simulink model "Mrinal_230929228_Simulink"  (R2025a)
settings: Solver=VariableStepAuto  StartTime=0.0  StopTime=40  RelTol=1e-3
libraries: spsSeriesRLCBranchLib x13, spsDCVoltageSourceLib x5, spsGroundLib x3, spsCurrentMeasurementLib x2, spsVoltageMeasurementLib x2, sps_lib x2
settings Model: Creator=MRINAL  LastModifiedBy=MRINAL

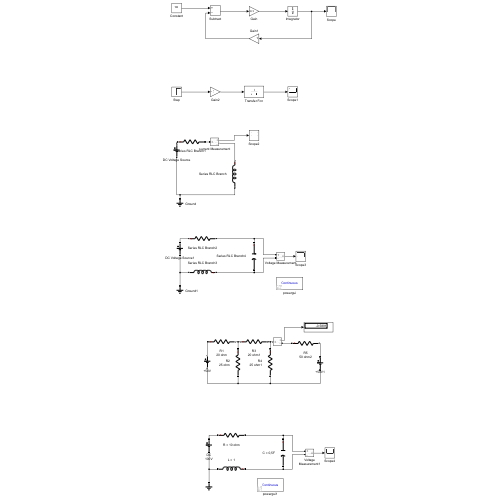
[thumbnail: Simulink's stored preview of the top-level diagram]
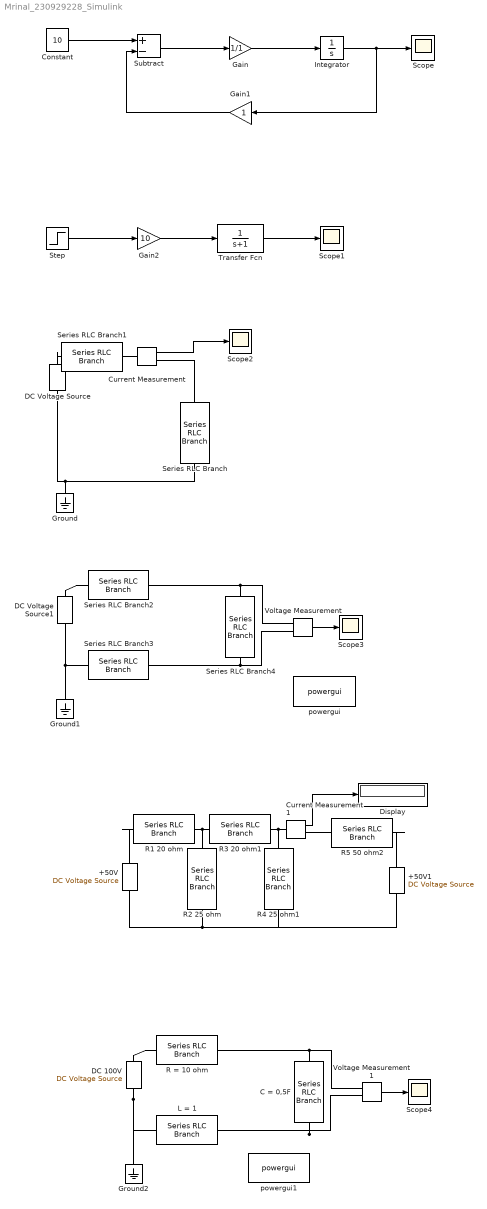
== system Mrinal_230929228_Simulink ==
  +50V : spsDCVoltageSourceLib/DC Voltage Source  Amplitude=50  Measurements=None
  +50V1 : spsDCVoltageSourceLib/DC Voltage Source  Amplitude=50  Measurements=None
  C = 0,5F : spsSeriesRLCBranchLib/Series RLC Branch  LConnTagsString=__new0  RConnTagsString=__new0  BranchType=C  Resistance=1  Inductance=1  SetiL0=off  InitialCurrent=0  Capacitance=0.5  Setx0=off  InitialVoltage=0  Measurements=None
  Constant : Constant  Value=10
  Current Measurement : spsCurrentMeasurementLib/Current Measurement  PhasorSimulation=off  OutputType=Complex  PSBequivalent=0
  Current Measurement1 : spsCurrentMeasurementLib/Current Measurement  PhasorSimulation=off  OutputType=Complex  PSBequivalent=0
  DC 100V : spsDCVoltageSourceLib/DC Voltage Source  Amplitude=100  Measurements=None
  DC Voltage Source : spsDCVoltageSourceLib/DC Voltage Source  Amplitude=10  Measurements=None
  DC Voltage Source1 : spsDCVoltageSourceLib/DC Voltage Source  Amplitude=10  Measurements=None
  Display : Display
  Gain : Gain  Gain=1/1
  Gain1 : Gain
  Gain2 : Gain  Gain=10
  Ground : spsGroundLib/Ground  LConnTagsString=a
  Ground1 : spsGroundLib/Ground  LConnTagsString=a
  Ground2 : spsGroundLib/Ground  LConnTagsString=a
  Integrator : Integrator
  L = 1 : spsSeriesRLCBranchLib/Series RLC Branch  LConnTagsString=__new0  RConnTagsString=__new0  BranchType=L  Resistance=1  Inductance=1  SetiL0=off  InitialCurrent=0  Capacitance=1e-6  Setx0=off  InitialVoltage=0  Measurements=None
  R = 10 ohm : spsSeriesRLCBranchLib/Series RLC Branch  LConnTagsString=__new0  RConnTagsString=__new0  BranchType=R  Resistance=1.23  Inductance=1e-3  SetiL0=off  InitialCurrent=0  Capacitance=1e-6  Setx0=off  InitialVoltage=0  Measurements=None
  R1 20 ohm : spsSeriesRLCBranchLib/Series RLC Branch  LConnTagsString=__new0  RConnTagsString=__new0  BranchType=R  Resistance=20  Inductance=1e-3  SetiL0=off  InitialCurrent=0  Capacitance=1e-6  Setx0=off  InitialVoltage=0  Measurements=None
  R2 25 ohm : spsSeriesRLCBranchLib/Series RLC Branch  LConnTagsString=__new0  RConnTagsString=__new0  BranchType=R  Resistance=25  Inductance=1e-3  SetiL0=off  InitialCurrent=0  Capacitance=1e-6  Setx0=off  InitialVoltage=0  Measurements=None
  R3 20 ohm1 : spsSeriesRLCBranchLib/Series RLC Branch  LConnTagsString=__new0  RConnTagsString=__new0  BranchType=R  Resistance=20  Inductance=1e-3  SetiL0=off  InitialCurrent=0  Capacitance=1e-6  Setx0=off  InitialVoltage=0  Measurements=None
  R4 25 ohm1 : spsSeriesRLCBranchLib/Series RLC Branch  LConnTagsString=__new0  RConnTagsString=__new0  BranchType=R  Resistance=25  Inductance=1e-3  SetiL0=off  InitialCurrent=0  Capacitance=1e-6  Setx0=off  InitialVoltage=0  Measurements=None
  R5 50 ohm2 : spsSeriesRLCBranchLib/Series RLC Branch  LConnTagsString=__new0  RConnTagsString=__new0  BranchType=R  Resistance=50  Inductance=1e-3  SetiL0=off  InitialCurrent=0  Capacitance=1e-6  Setx0=off  InitialVoltage=0  Measurements=None
  Scope{,1..4} (5 alike) : Scope
      Scope settings: Title=230929228_Mrinal_Kumar  ActiveDisplayYMinimum=-1  ActiveDisplayYMaximum=1  YLabel=Current
      Scope1 settings: Title=230929228_Mrinal_Kumar  ActiveDisplayYMinimum=-1.2498457375731515  ActiveDisplayYMaximum=11.248611638158366  YLabel=Current
      Scope2 settings: Title=230929228_Mrinal_Kumar  ActiveDisplayYMinimum=-1  ActiveDisplayYMaximum=1  DataLoggingVariableName=ScopeData2
      Scope3 settings: Title=230929228_Mrinal_Kumar  ActiveDisplayYMinimum=-1.2499701795989464  ActiveDisplayYMaximum=11.24973161639052  YLabel=Voltage (V)  DataLoggingVariableName=ScopeData3
      Scope4 settings: Title=230929228_Mrinal_Kumar  ActiveDisplayYMinimum=-14.98597735302806  ActiveDisplayYMaximum=134.87379617725259  YLabel=Voltage (V)  DataLoggingVariableName=ScopeData4
  Series RLC Branch : spsSeriesRLCBranchLib/Series RLC Branch  LConnTagsString=__new0  RConnTagsString=__new0  BranchType=L  Resistance=1  Inductance=1  SetiL0=off  InitialCurrent=0  Capacitance=1e-6  Setx0=off  InitialVoltage=0  Measurements=None
  Series RLC Branch1 : spsSeriesRLCBranchLib/Series RLC Branch  LConnTagsString=__new0  RConnTagsString=__new0  BranchType=R  Resistance=1  Inductance=1e-3  SetiL0=off  InitialCurrent=0  Capacitance=1e-6  Setx0=off  InitialVoltage=0  Measurements=None
  Series RLC Branch2 : spsSeriesRLCBranchLib/Series RLC Branch  LConnTagsString=__new0  RConnTagsString=__new0  BranchType=R  Resistance=4  Inductance=1e-3  SetiL0=off  InitialCurrent=0  Capacitance=1e-6  Setx0=off  InitialVoltage=0  Measurements=None
  Series RLC Branch3 : spsSeriesRLCBranchLib/Series RLC Branch  LConnTagsString=__new0  RConnTagsString=__new0  BranchType=L  Resistance=1  Inductance=1  SetiL0=off  InitialCurrent=0  Capacitance=1e-6  Setx0=off  InitialVoltage=0  Measurements=None
  Series RLC Branch4 : spsSeriesRLCBranchLib/Series RLC Branch  LConnTagsString=__new0  RConnTagsString=__new0  BranchType=C  Resistance=1  Inductance=1  SetiL0=off  InitialCurrent=0  Capacitance=1  Setx0=off  InitialVoltage=0  Measurements=None
  Step : Step  SampleTime=0
  Subtract : Sum  Inputs=+-
  Transfer Fcn : TransferFcn  Denominator=[1 1]
  Voltage Measurement1 : spsVoltageMeasurementLib/Voltage Measurement  PhasorSimulation=off  OutputType=Complex  PSBequivalent=0
  Voltage Measurement : spsVoltageMeasurementLib/Voltage Measurement  PhasorSimulation=off  OutputType=Complex  PSBequivalent=0
  powergui : sps_lib/powergui  Priority=1  SimulationMode=Continuous  SampleTime=50e-6  frequency=60  Iterations=50  frequencyindice=0  Pbase=100e6  ErrMax=1e-4  UnitsV=kV  UnitsW=MW  buscounter=0  FunctionMessages=off  echomessages=off  EnableUseOfTLC=off  CurrentSourceSwitches=off  DisableSnubberDevices=off  DisableRonSwitches=off  DisableVfSwitches=off  DisplayEquations=off  AutomaticDiscreteSolvers=off  SolverType=Tustin/Backward Euler (TBE)  Interpol=off  ExternalGateDelay=off  methode=off  Ts=100  x0status=zero  SPID=on  SwTol=0  HookPort=off  NonlinearTolerance=1e-4  nMaxIteration=100  ContinueOnMaxIteration=off  RestoreLinks=warning  ResistiveCurrentMeasurement=off  Frange=[0:2:500]  Ylog=off  Xlog=on  ShowGrid=off  save=off  variable=ZData  structure=0  ZoomFFT=off  StartTime=0.0  cycles=1  DisplayStyle=1  fundamental=60  FreqAxis=off  MaxFrequency=1000  frequencyindicesteady=1  RmsSteady=1  display=off
  powergui1 : sps_lib/powergui  Priority=1  SimulationMode=Continuous  SampleTime=50e-6  frequency=60  Iterations=50  frequencyindice=0  Pbase=100e6  ErrMax=1e-4  UnitsV=kV  UnitsW=MW  buscounter=0  FunctionMessages=off  echomessages=off  EnableUseOfTLC=off  CurrentSourceSwitches=off  DisableSnubberDevices=off  DisableRonSwitches=off  DisableVfSwitches=off  DisplayEquations=off  AutomaticDiscreteSolvers=off  SolverType=Tustin/Backward Euler (TBE)  Interpol=off  ExternalGateDelay=off  methode=off  Ts=100  x0status=zero  SPID=on  SwTol=0  HookPort=off  NonlinearTolerance=1e-4  nMaxIteration=100  ContinueOnMaxIteration=off  RestoreLinks=warning  ResistiveCurrentMeasurement=off  Frange=[0:2:500]  Ylog=off  Xlog=on  ShowGrid=off  save=off  variable=ZData  structure=0  ZoomFFT=off  StartTime=0.0  cycles=1  DisplayStyle=1  fundamental=60  FreqAxis=off  MaxFrequency=1000  frequencyindicesteady=1  RmsSteady=1  display=off
  wires:
  Constant/1 -> Subtract/1
  Subtract/1 -> Gain/1
  Gain/1 -> Integrator/1
  Integrator/1 -> Gain1/1, Scope/1
  Gain1/1 -> Subtract/2
  Step/1 -> Gain2/1
  Gain2/1 -> Transfer Fcn/1
  Transfer Fcn/1 -> Scope1/1
  Current Measurement/1 -> Scope2/1
  Voltage Measurement/1 -> Scope3/1
  Current Measurement1/1 -> Display/1
  Voltage Measurement1/1 -> Scope4/1
  connections:
  Current Measurement/RConn1 -- Series RLC Branch/LConn1
  Series RLC Branch/RConn1 -- DC Voltage Source/LConn1 -- Ground/LConn1
  DC Voltage Source/RConn1 -- Series RLC Branch1/LConn1
  Series RLC Branch1/RConn1 -- Current Measurement/LConn1
  Ground1/LConn1 -- Series RLC Branch3/RConn1 -- DC Voltage Source1/LConn1
  Series RLC Branch2/LConn1 -- DC Voltage Source1/RConn1
  Series RLC Branch4/LConn1 -- Series RLC Branch2/RConn1 -- Voltage Measurement/LConn1
  Series RLC Branch3/LConn1 -- Voltage Measurement/LConn2 -- Series RLC Branch4/RConn1
  R3 20 ohm1/LConn1 -- R2 25 ohm/LConn1 -- R1 20 ohm/RConn1
  R4 25 ohm1/LConn1 -- Current Measurement1/LConn1 -- R3 20 ohm1/RConn1
  R1 20 ohm/LConn1 -- +50V/RConn1
  R2 25 ohm/RConn1 -- +50V1/LConn1 -- R4 25 ohm1/RConn1 -- +50V/LConn1
  R5 50 ohm2/RConn1 -- +50V1/RConn1
  Current Measurement1/RConn1 -- R5 50 ohm2/LConn1
  C = 0,5F/RConn1 -- L = 1/LConn1 -- Voltage Measurement1/LConn2
  Voltage Measurement1/LConn1 -- C = 0,5F/LConn1 -- R = 10 ohm/RConn1
  DC 100V/LConn1 -- Ground2/LConn1 -- L = 1/RConn1
  R = 10 ohm/LConn1 -- DC 100V/RConn1
